simulink model "EMC_gaze"  (R2015a)
settings: Solver=ode4  SolverMode=MultiTasking  StartTime=0.0  StopTime=inf  FixedStep=BKIN_STEP_TIME  RelTol=1e-3
StartFcn:
  |  warndlg('Dexterit-E models cannot run under simulation. Please compile your model and run it from within Dexterit-E.');set_param(bdroot,'SimulationCommand','stop')
model workspace (MAT data in the model file):
  BKIN_KINEMATIC_FRAME_SIZE = 400
  BKIN_STEP_TIME = 0.00025
  COLOR = 4
  COL_X = 1
  COL_Y = 2
  E_NO_EVENT = 0
  LOAD_X = 1
  LOAD_Y = 2
  MOVEMENT_DELAY = 3
  PATH_LENGTH = 1
  PATH_PERIOD = 2
  POST_TRIAL_DELAY = 4
  RADIUS = 3
  TRAJECTORY = 1
  TRAJECTORY_TYPE = 2
  TRIAL_END = 3
  TRIAL_MOVEMENT = 2
  TRIAL_RESET = 4
  TRIAL_START = 1
  X_POSITION = 1
  Y_POSITION = 2
  col_x = 1
  col_y = 2
  ANGULAR_THRESHOLD = 5
  GAZE_EXIT = 6
  START_REACHED = 7
  FIXATION_DURATION = 6
  TRACKING_TARGET_ROW = 7
  FEEDBACK_COLOR = 5
  CROSS_LOGICAL_RADIUS = 8
  DETECT_FIXATION = 8
  GAZE_IN_TARGET = 5
  START_STABILIZATION = 9
  HAND_IN_TARGET = 9
  BACKGROUND_LOAD = 10
  DIST_BETWEEN_TRAJ = 11
  STRAIGHT_PAUSE_TIME = 12
libraries: simulink x14, xpcrtudplib x12, xpcutilitieslib x10, xpcobsoletelib x8, slrtlib x2, ethercat x2, General x2, Video x2, KINARM_EP_loads x1, KINARM_general x1
(part 5 of 7)

== matlab function EMC_gaze/DataLogging/Receive_Gaze/Embedded MATLAB Function1 ==
  data: input input; pupil_area_PIXELS input; tracking_status input; tracking_available input; camtheta input; camera_GLOBAL input; focal_length input; gazeXYCalculated output; head_data input; pupil_area_GLOBAL output; gaze_unit_vector_GLOBAL output; pupil_GLOBAL output; target_GLOBAL output
function [gazeXYCalculated, pupil_area_GLOBAL, gaze_unit_vector_GLOBAL, pupil_GLOBAL, target_GLOBAL] = fcn(input, pupil_area_PIXELS, tracking_status, tracking_available, camtheta,camera_GLOBAL, focal_length, head_data)

% The following are some details on the Eyelink camera
EL_target_distance_scaling_factor = 10000;					%target distance is reported by Eyelink in 1/10 of mm units
EL_pix_per_mm = 200;										%there are 200 pixels/mm on the Eyelink 1000 camera sensor

raw_pupil = [input(1) input(2)];
href = [input(3); input(4); 0];
target_distance_in = head_data(3);
%%%%%%%%%%%%%%%%%%%%%%%%%%%%%%%%%%
%% Tarkesh
target_position_in = head_data(1:2);
%%%%%%%%%%%%%%%%%%%%%%%%%%%%%%%%%%%%%%
target_distance = target_distance_in / EL_target_distance_scaling_factor;		% distance of the target from the camera (m)

%if there is a blink or other problem then send out errors. C3D file does not like NaN, so we output -100.
if tracking_status == 4 || tracking_available == 0 || (href(1) == 0 && href(2) == 0) || (raw_pupil(1) == -32768 && raw_pupil(2) == -32768)
    gazeXYCalculated = [-100; -100];
	pupil_area_GLOBAL = -100;
    gaze_unit_vector_GLOBAL = [-100; -100; -100];
    pupil_GLOBAL = [-100; -100; -100];
    target_GLOBAL = [-100; -100; -100];
    return
end

[Rx Ry Rz] = calc_R_from_angles(camtheta(1), camtheta(2), 0);
R_CMRA2GLBL = Rx * Ry;
%R_GLBL2CMRA = R_CMRA2GLBL';

%camera_GLOBAL_Trans = camera_GLOBAL';
pupil_XY_Sensor = convertPupilToSensor(raw_pupil(1), raw_pupil(2), EL_pix_per_mm);
[gaze_GLOBAL, pupil_GLOBAL] = calc_GAZE(pupil_XY_Sensor, target_distance, href, focal_length, camera_GLOBAL, R_CMRA2GLBL);
gazeXYCalculated = gaze_GLOBAL(1:2);

%%%%%%%%%%%%%%%%%%%%%%%%%%5
%% Tarkesh
target_XY_Sesor = convertPupilToSensor(target_position_in(1), target_position_in(2), EL_pix_per_mm);
[~, target_GLOBAL] = calc_GAZE(target_XY_Sesor, target_distance, href, focal_length, camera_GLOBAL, R_CMRA2GLBL);
%%%%%%%%%%%%%%%%%%%%%%%%%%

%%convert the pupil area from pixels on the sensor, to m^2, correcting for camera and gaze angle
% pupil area on the camera sensor, in m^2
pupil_area_SENSOR = pupil_area_PIXELS / ( (EL_pix_per_mm * 1000 ) ^ 2);		

% pupil area in the global workspace, projected onto a plane parallel to the camera sensor in m^2
pupil_area_GLOBAL_projection = pupil_area_SENSOR * (target_distance / focal_length) ^ 2; 

% create a unit vector that is normal to the camera sensor, in GLOBAL coordinates
sensor_unit_vector_GLOBAL = R_CMRA2GLBL * [0; 0; 1];

% create a unit vector for the subject's gaze
gaze_vector_GLOBAL = pupil_GLOBAL - gaze_GLOBAL;
gaze_unit_vector_GLOBAL = gaze_vector_GLOBAL / norm(gaze_vector_GLOBAL);

% calculate the cosine of the angle between the unit vectors for gaze and the camera sensor
cos_gaze_camera_angle = dot(sensor_unit_vector_GLOBAL, gaze_unit_vector_GLOBAL); 

% correct the pupil area to account for the angle of the eye relative to the camera sensor plane
% We assume that the pupil is circular. In the plane formed by the two vectors, the distance needs 
% to be scaled by cos(theta). In the perpendicular plane, there is no scaling. Hence we do NOT 
% square the cos(theta) and the area is only corrected for by 1 / cos(theta). 
pupil_area_GLOBAL = pupil_area_GLOBAL_projection / cos_gaze_camera_angle;

% % % % For testing
% % % gaze_camera_angle  = acos(cos_gaze_camera_angle) * 180/pi();
% % % HREF_angle = atan2( norm(href), 15000) * 180 / pi();
% % % testing = [pupil_area_SENSOR*1e6, pupil_area_GLOBAL_projection*1e6, pupil_area_GLOBAL*1e6, gaze_camera_angle, HREF_angle, cos_gaze_camera_angle];
% % % testing2 = [sensor_unit_vector_GLOBAL; gaze_unit_vector_GLOBAL];



%% Functions
function [gaze_est_GLOBAL, pupil_GLOBAL] = calc_GAZE(pupil_SENSOR, target_distance, HREF_HREF, focal_length, camera_GLOBAL, R_CMRA2GLBL)
    % This function estimates GAZE based on data from the Eyelink.  To be used
    % during 'running' of a task. 

    % Convert pupil location from Eyelink sensor frame to camera reference
    % frame with camera at origin and rotated to camera's angle (W-axis along
    % camera's point of view)  
    pupil_CAMERA = [pupil_SENSOR * target_distance / focal_length; target_distance];
    pupil_distance = norm(pupil_CAMERA);

    % Rotation matrix to convert from HREF coordinates to camera coordinates.
    % HREF z-axis is defined as ray from camera to pupil.
    R_HREF2CMRA = calc_R_from_vectors(pupil_CAMERA, [0; 0; 1]);

    % Convert the HREF from HREF coordinates to canera coordinates.  Scale,
    % then rotate. 
    HREF_CAMERA = R_HREF2CMRA * (HREF_HREF * pupil_distance / 15000);

    % Then convert pupil and HREF locations from camera frame to global frame
    % by rotating and then shifting origins. 
    pupil_GLOBAL = R_CMRA2GLBL * pupil_CAMERA + camera_GLOBAL';
    HREF_GLOBAL = R_CMRA2GLBL * HREF_CAMERA + camera_GLOBAL';

    % Find intersection of gaze_ray (from pupil to HREF) with the subject_display plane
    norm_vector = [0; 0; 1];		% In the KINARM VR setup, the Z-axis is defined as normal to the subject display
    point_on_plane = [0; 0; 0];		% In the KINARM VR setup, the origin is defined as on the subject display plane

    % display([pupil_GLOBAL HREF_GLOBAL])
    gaze_est_GLOBAL = plane_line_intersect(norm_vector, point_on_plane, pupil_GLOBAL, HREF_GLOBAL);

function pupil_XY_Sensor = convertPupilToSensor(pupilX, pupilY, pix_per_mm)
%         Returns the projection of the pupil on the camera sensor in meters, based on inputs in some raw unit (not pixels)

    % the following constants are from Jiye, email Nov 7, 2011
    LEFTDROP = 32;				%pixels dropped at left of sensor
    TOPDROP = 48;				%lines dropped at top of sensor
    const_x = 7*176;			%no idea what this is.  Maybe number of pixels???
    const_y = 4*184 + 188;		%no idea what this is.  Maybe number of pixels???

    % from Jiye. Not sure excatly what they are (probably camera center in pixels)
    cam_rot_cx = const_x / 2 + LEFTDROP;			
    cam_rot_cy = const_y / 2 +TOPDROP;

    hor = 30000;
    lor = -30000;
    hr = 0.9;
    lr = 0.1;
    ld = 50;
    hdx = 1200;		%hmmm almost same as const_x, which is 1232
    hdy = 920;		%hmmm almost same as const_y, which is 924

    scx = (hor-lor) / (hdx - ld) / (hr-lr);
    ofx = lor - (ld + (hdx - ld) * lr )* scx;

    scy = (hor-lor) / (hdy - ld) / (hr-lr);
    ofy = lor - (ld + (hdy - ld) * lr )* scy;

    % calculate the pupil in camera sensor coordinates (pixels)
    px = (pupilX - ofx) / scx;
    py = (pupilY - ofy) / scy;

    ppl_mmX = - ( (cam_rot_cx - px) / pix_per_mm );
    ppl_mmY =   ( (cam_rot_cy - py) / pix_per_mm );

    pupil_XY_Sensor = [ppl_mmX / 1000; ppl_mmY / 1000];
    
function [Rx Ry Rz] = calc_R_from_angles(xrot, yrot, zrot)
    % This function creates the three rotation matrices for rotations about the
    % x, y and z axes.  Input rotations are in degrees.

    xrot = xrot/180*pi;		%convert to radians
    yrot = yrot/180*pi;		%convert to radians
    zrot = zrot/180*pi;		%convert to radians
    Rx = [1 0 0; 0 cos(xrot) -sin(xrot); 0 sin(xrot) cos(xrot)]; 
    Ry = [cos(yrot) 0 sin(yrot); 0 1 0; -sin(yrot) 0 cos(yrot)]; 
    Rz = [cos(zrot) -sin(zrot) 0; sin(zrot) cos(zrot) 0 ; 0 0 1]; 

    
function R = calc_R_from_vectors(v1, v2)
    % This function calculates a rotation matrix, given two vectors, such that
    % the rotation matrix will rotate from v1 to v2.

    rot_axis = cross(v2, v1);			%axis that is perpendicular to the two vectors

    % If either of the vectors v1 or v2 is = [0 0 0], or if they are parallel
    % (i.e. norm(rot_axis) == 0), then there is no rotation.  But math errors
    % will occur, so we need to check for these cases.   
    if (norm(v1) == 0) || (norm(v2) == 0)	|| (norm(rot_axis) == 0)
        R = eye(3);																%identity matrix results in no rotation
    else
        rot_angle = asin( norm(rot_axis) / norm(v1) / norm(v2) );				%angle of rotation about rot_axis
        n = rot_axis / norm(rot_axis);											%normalize to get a unit vector for the rotation
        n_cross_product_matrix = [ 0 -n(3) n(2); n(3) 0 -n(1); -n(2) n(1) 0];	%def'n of cross product matrix
        cosA = cos(rot_angle);
        sinA = sin(rot_angle);
        R = eye(3) * cosA + sinA * n_cross_product_matrix + (1 - cosA) * (n * n');
    % 	display(rot_angle);
    end


function I = plane_line_intersect(n,V0,P0,P1)
    %plane_line_intersect computes the intersection of a plane and a segment(or
    %a straight line)
    % Inputs: 
    %       n: normal vector of the Plane 
    %       V0: any point that belongs to the Plane 
    %       P0: end point 1 of the segment P0P1
    %       P1:  end point 2 of the segment P0P1
    %
    %Outputs:
    %      I    is the point of interection 
    %     Check is (DELETED AND NOT USED HERE) an indicator:
    %      0 => disjoint (no intersection)
    %      1 => the plane intersects P0P1 in the unique point I
    %      2 => the segment lies in the plane
    %      3=>the intersection lies outside the segment P0P1
    %
    % Example:
    % Determine the intersection of following the plane x+y+z+3=0 with the segment P0P1:
    % The plane is represented by the normal vector n=[1 1 1]
    % and an arbitrary point that lies on the plane, ex: V0=[1 1 -5]
    % The segment is represented by the following two points
    % P0=[-5 1 -1]
    %P1=[1 2 3]   
    % [I,check]=plane_line_intersect([1 1 1],[1 1 -5],[-5 1 -1],[1 2 3]);

    %This function is written by :
    %                             Nassim Khaled
    %                             Wayne State University
    %                             Research Assistant and Phd candidate
    %If you have any comments or face any problems, please feel free to leave
    %your comments and i will try to reply to you as fast as possible.

    I=[0; 0; 0];
    u = P1-P0;
    w = P0 - V0;
    D = dot(n,u);
    N = -dot(n,w);
    check=0;
    if abs(D) < 10^-7        % The segment is parallel to plane
            if N == 0           % The segment lies in plane
                check=2;
                return
            else
                check=0;       %no intersection
                return
            end
    end

    %compute the intersection parameter
    sI = N / D;
    I = P0+ sI.*u;

== matlab function EMC_gaze/DataLogging/Receive_Gaze/clean_packet ==
  data: pack_in input; pack_out output; len_out output; len_in input
function [pack_out, len_out] = clean_packet(pack_in, len_in)

%for some reason, during calibration we can get very large packets that 
%blow up the c code for parsing the packets. If we get a large packet
%we can ignore it.

if len_in < 512
    pack_out = pack_in;
    len_out = len_in;
else
    pack_out = zeros(512, 1, 'uint8');
    len_out = int32(0);
end

== matlab function EMC_gaze/DataLogging/Receive_Gaze/convert to seconds2 ==
  data: event_data input; event_data_out output; start_time input; eyelink_timestamp input
function event_data_out = fcn(event_data, start_time, eyelink_timestamp)

persistent last_timestamp

if isempty(last_timestamp)
	last_timestamp = uint32(0);
end

%DEX-3313 if eyelink has stopped sending us data then we should not flood
%Dex with events.
if last_timestamp == eyelink_timestamp
	event_data_out = [0; 0; 0];
	return
end

last_timestamp = eyelink_timestamp;
event_data_out = event_data;

if event_data(1) ~= 0
    event_data_out(2) = (event_data(2) - start_time) / 1000.0;
    event_data_out(3) = (event_data(3) - start_time) / 1000.0;
end

== matlab function EMC_gaze/KINARM_EP_Apply_Loads/Remove_NaNs_and_Inf ==
  settings: fimath=|
      | fimath(...
      | 'RoundMode', 'floor',...
      | 'OverflowMode', 'wrap',...
      | 'ProductMode', 'KeepLSB', 'ProductWordLength', 32,...
      | 'SumMode', 'KeepLSB', 'SumWordLength', 32,...
      | 'CastBeforeSum', false)
  data: in input; out output
function out= fcn(in)

% This function removes all infinite and NaN values from the input.

out = zeros(size(in));		%default value of output

for ii = 1:length(in)
	if isfinite( in(ii) )	%only pass the input to the output if it is finite
		out(ii) = in(ii); 
	end
end

== matlab function EMC_gaze/KINARM_EP_Apply_Loads/Remove_NaNs_and_Inf1 ==
  settings: fimath=|
      | fimath(...
      | 'RoundMode', 'floor',...
      | 'OverflowMode', 'wrap',...
      | 'ProductMode', 'KeepLSB', 'ProductWordLength', 32,...
      | 'SumMode', 'KeepLSB', 'SumWordLength', 32,...
      | 'CastBeforeSum', false)
  data: in1 input; out output; in2 input; in3 input; in4 input
function out= fcn( in1,in2,in3,in4)

% This function removes all infinite and NaN values from the input.

out = [in1 in2 in3 in4];
if ~isfinite(in1)
    out(1) = 0;
end
if ~isfinite(in2)
    out(2) = 0;
end
if ~isfinite(in3)
    out(3) = 0;
end
if ~isfinite(in4)
    out(4) = 0;
end

== matlab function EMC_gaze/KINARM_EP_Apply_Loads/detect motor state/MATLAB Function ==
  data: motor_status input; motors_enabled output; grip_sensor input; is_ecat input
function motors_enabled = fcn(motor_status, grip_sensor, is_ecat)
%#codegen

motors_enabled = motor_status == 0 && (~is_ecat || grip_sensor == 1);

== matlab function EMC_gaze/KINARM_EP_Apply_Loads/detect motor state1/MATLAB Function ==
  data: motor_status input; motors_enabled output; grip_sensor input; is_ecat input
function motors_enabled = fcn(motor_status, grip_sensor, is_ecat)
%#codegen

motors_enabled = motor_status == 0 && (~is_ecat || grip_sensor == 1);

== matlab function EMC_gaze/DataLogging/Poll Force Plates/plate1/parse packet 1 ==
  data: packet input; forces output; moments output; timer output; calibration input; gain input; ain_slope input; ain_offset input; orientation input; zero_voltage input
function [forces, moments, timer] = fcn(packet, calibration, gain, ain_slope, ain_offset, orientation, zero_voltage)
    %This pulls voltages and timer infomation from the packet we got back from
    %the lab jack.
    
    voltages = zeros(1, 8);
    timers = zeros(1, 3);
    
    for n = 1:8
        bits = readUShort(packet, 13 + ((n - 1)*2));
        voltages(n) = binaryToCalibratedAnalogVoltage(bits, ain_slope, ain_offset);
    end
    
    for n = 1:3
        timers(n) = readUInt(packet, 53 + ((n - 1)*4));
    end
    
    %convert the time stamp to a time in seconds.
    timer = timers(1) / 750000.0; 
    
    %all voltages are between -2.5 to 2.5, here we are normalizeing what we read to zero.
    voltages = voltages - zero_voltage;
    voltages = voltages(1:8); % only the first 8 channels matter.
    
    %using the calibration matrix we convert the to the forces and moments
    values = calibration * (voltages / gain)';
    forces = values(1:3);
    moments = values(4:6);
    
	%reverse the Z force to get it into global coordinates.
	forces(3) = -forces(3);
	
	%considering the positions of the cables push all measures into global coordinates
    if orientation == 0
        forces(2) = -forces(2);
        moments(2) = -moments(2);
    elseif orientation == 90
        y = forces(2);
        forces(2) = -forces(1);
        forces(1) = -y;

        y = moments(2);
        moments(2) = -moments(1);
        moments(1) = -y;
	elseif orientation == 180
        forces(1) = -forces(1);        
        moments(1) = -moments(1);        
    elseif orientation == 270
        y = forces(2);
        forces(2) = forces(1);
        forces(1) = y;

		y = moments(2);
        moments(2) = moments(1);
        moments(1) = y;
    end
end

function val = readUShort(data, offset)
    p1 = uint32(data(offset));
    p2 = uint32(data(offset + 1));
    val = double(p1 + (p2 * 256));
end

function val = readUInt(data, offset)
    p1 = uint32(data(offset));
    p2 = uint32(data(offset + 1));
    p3 = uint32(data(offset + 2));
    p4 = uint32(data(offset + 3));
    val = double(p1 + (p2 * 256) + (p3 * 2^16) + (p4 * 2^24));
end

function voltage = binaryToCalibratedAnalogVoltage(bits, ain_slope, ain_offset)
    voltage = (bits * ain_slope) + ain_offset;
end

== matlab function EMC_gaze/DataLogging/Poll Force Plates/plate2/parse packet 1 ==
  data: packet input; forces output; moments output; timer output; calibration input; gain input; ain_slope input; ain_offset input; orientation input; zero_voltage input
function [forces, moments, timer] = fcn(packet, calibration, gain, ain_slope, ain_offset, orientation, zero_voltage)
    %This pulls voltages and timer infomation from the packet we got back from
    %the lab jack.
    
    voltages = zeros(1, 8);
    timers = zeros(1, 3);

    for n = 1:8
        bits = readUShort(packet, 13 + ((n - 1)*2));
        voltages(n) = binaryToCalibratedAnalogVoltage(bits, ain_slope, ain_offset);
    end
    
    for n = 1:3
        timers(n) = readUInt(packet, 53 + ((n - 1)*4));
    end
    
    %convert the time stamp to a time in seconds.
    timer = timers(1) / 750000.0; 
    
    %all voltages are between -2.5 to 2.5, here we are normalizeing what we read to zero.
    voltages = voltages - zero_voltage;
    voltages = voltages(1:8); % only the first 8 channels matter.
    
    %using the calibration matrix we convert the to the forces and moments
    values = calibration * (voltages / gain)';
    forces = values(1:3);
    moments = values(4:6);
    
	%reverse the Z force to get it into global coordinates.
	forces(3) = -forces(3);

	%considering the positions of the cables push all measures into global coordinates
    if orientation == 0
        forces(2) = -forces(2);
        moments(2) = -moments(2);
    elseif orientation == 90
        y = forces(2);
        forces(2) = -forces(1);
        forces(1) = -y;

        y = moments(2);
        moments(2) = -moments(1);
        moments(1) = -y;
	elseif orientation == 180
        forces(1) = -forces(1);        
        moments(1) = -moments(1);        
    elseif orientation == 270
        y = forces(2);
        forces(2) = forces(1);
        forces(1) = y;

		y = moments(2);
        moments(2) = moments(1);
        moments(1) = y;
    end
end

function val = readUShort(data, offset)
    p1 = uint32(data(offset));
    p2 = uint32(data(offset + 1));
    val = double(p1 + (p2 * 256));
end

function val = readUInt(data, offset)
    p1 = uint32(data(offset));
    p2 = uint32(data(offset + 1));
    p3 = uint32(data(offset + 2));
    p4 = uint32(data(offset + 3));
    val = double(p1 + (p2 * 256) + (p3 * 2^16) + (p4 * 2^24));
end

function voltage = binaryToCalibratedAnalogVoltage(bits, ain_slope, ain_offset)
    voltage = (bits * ain_slope) + ain_offset;
end

== matlab function EMC_gaze/DataLogging/Poll KINARM/Force Sensor Control/Force Sensor 1 Subsystem/Create timestamp ==
  data: times_in input; timestamp_out output
function timestamp_out = fcn(times_in)

persistent start_time
persistent last_time

if isempty(start_time)
   start_time = uint32(0);
end

if isempty(last_time)
    last_time = uint32(0);
end

if start_time == 0 && times_in(2) > 0
    start_time = times_in(2);
end

if times_in(2) < start_time
    start_time = -(last_time - start_time);
end

%F/T sensor clock runs at 7Khz according to the manual,
%using a 32 bit integer for this gives about 7 days before it will roll
%over. This means we need to account for roll overs in order to make
%analysis sane.
timestamp_out = double(times_in(2) - start_time) / 7000.0;
last_time = times_in(2);

== matlab function EMC_gaze/DataLogging/Poll KINARM/Force Sensor Control/Force Sensor 2 Subsystem/Create timestamp ==
  data: times_in input; timestamp_out output
function timestamp_out = fcn(times_in)

persistent start_time
persistent last_time

if isempty(start_time)
   start_time = uint32(0);
end

if isempty(last_time)
    last_time = uint32(0);
end

if start_time == 0 && times_in(2) > 0
    start_time = times_in(2);
end

if times_in(2) < start_time
    start_time = -(last_time - start_time);
end

%F/T sensor clock runs at 7Khz according to the manual,
%using a 32 bit integer for this gives about 7 days before it will roll
%over. This means we need to account for roll overs in order to make
%analysis sane.
timestamp_out = double(times_in(2) - start_time) / 7000.0;
last_time = times_in(2);

== matlab function EMC_gaze/DataLogging/Poll KINARM/PMAC Subsystem/read_pmac/DPRAM Access Subsystem/TypeCast ==
  data: u input; y output
function y = fcn(u)

% EML determines output class and size based on first usage
% for some reason the typecast is not setting it correctly, so we 
% explicitly define it first.
y = single(0);

% in order for the typecast to work, both temp and y must be 32 bit
temp = cast(u, 'uint32');
y = typecast(temp, 'single');

== matlab function EMC_gaze/DataLogging/Poll KINARM/PMAC Subsystem/read_pmac/Monitor_status ==
  data: status_data input; servo_counter input; robotCount input; force_scale output; plcc_version input
function force_scale = monitor_system_status(status_data, servo_counter, robotCount, plcc_version)

persistent no_update_count;
persistent last_servo_counter;

if isempty(no_update_count)
   no_update_count = 0;
end

if isempty(last_servo_counter)
    last_servo_counter = uint32(0);
end

pmac_fault_state = uint32(status_data(2));
plcc_switch = status_data(3);
force_scale = 1;

%plcc versions >1000 are custom
if plcc_version >= 6.0 && plcc_version < 1000
    %if the task is running and the servo amp counter is not
    if plcc_switch == 4.0 && last_servo_counter == servo_counter
        no_update_count = no_update_count + 1;    
        %after 5 cycles with the counter not running we should kill forces.
        if no_update_count >= 5
            force_scale = 0;
        end
    else
        no_update_count = 0;
    end
    last_servo_counter = servo_counter; 
end

%plcc versions >1000 are custom
if plcc_version >= 7.0 && plcc_version < 1000
    %if it is unilateral and the robot state is faulted then kill the forces
    if robotCount == 1 && bitand(pmac_fault_state, 1) == 1
        force_scale = 0;
    %if the system is bilateral and either robot is faulted, kill forces.
    elseif robotCount == 2 && bitand(pmac_fault_state, 3) ~= 0
        force_scale = 0;
    end
end

if plcc_version == 0
    force_scale = 0;
end

== matlab function EMC_gaze/DataLogging/Poll KINARM/PMAC Subsystem/read_pmac/Robot_data_builder ==
  data: bR1HasSecondardy input; bR2HasSecondardy input; robot1Data input; robot2Data input; robot1PrimaryEncData input; robot2PrimaryEncData input; robot1DataOut output; robot2DataOut output; servoCounter input; plccVer input; robot1PrimaryEncDataOut output; robot2PrimaryEncDataOut output
function [robot1DataOut, robot2DataOut, robot1PrimaryEncDataOut, robot2PrimaryEncDataOut] = convertPMACValues(bR1HasSecondardy, bR2HasSecondardy, robot1Data, robot2Data, robot1PrimaryEncData, robot2PrimaryEncData, servoCounter, plccVer)

    persistent robot1Struct robot2Struct robot1StructPrimary robot2StructPrimary servoValuesR1 servoValuesR2
    
    if isempty(robot1Struct)
        robot1Struct = getStruct();
        robot2Struct = getStruct();
        robot1StructPrimary = getStruct();
        robot2StructPrimary = getStruct();
        servoValuesR1 = zeros(5, 1);
        servoValuesR2 = zeros(5, 1);
    end
    
    if plccVer < 7
        robot1DataOut = robot1Data;
        robot2DataOut = robot2Data;
        robot1PrimaryEncDataOut = robot1PrimaryEncData;
        robot2PrimaryEncDataOut = robot2PrimaryEncData;
        return
    end
    
    if servoCounter(1) ~= servoValuesR1(1)
        robot1Struct = updatePositions(robot1Struct, robot1Data, bR1HasSecondardy);
        robot1StructPrimary = updatePositions(robot1StructPrimary, robot1PrimaryEncData, 0);
        servoValuesR1 = insertVal(servoValuesR1, servoCounter(1));
        robot1Struct = calculateVelAcc(robot1Struct, servoValuesR1, robot1Data);
        robot1StructPrimary = calculateVelAcc(robot1StructPrimary, servoValuesR1, robot1PrimaryEncData);
    end
    
    if servoCounter(2) ~= servoValuesR2(1)
        robot2Struct = updatePositions(robot2Struct, robot2Data, bR2HasSecondardy);
        robot2StructPrimary = updatePositions(robot2StructPrimary, robot2PrimaryEncData, 0);
        servoValuesR2 = insertVal(servoValuesR2, servoCounter(2));
        robot2Struct = calculateVelAcc(robot2Struct, servoValuesR2, robot2Data);
        robot2StructPrimary = calculateVelAcc(robot2StructPrimary, servoValuesR2, robot2PrimaryEncData);
    end
    
    robot1DataOut = insertVelAcc(robot1Data, robot1Struct);
    robot2DataOut = insertVelAcc(robot2Data, robot2Struct);

    robot1PrimaryEncDataOut = insertVelAcc(robot1PrimaryEncData, robot1StructPrimary);
    robot2PrimaryEncDataOut = insertVelAcc(robot2PrimaryEncData, robot2StructPrimary);
    
    %We used to provide a filtered velocity, but we can't with EtherCAT and
    %it was not being used anywhere anyway. 
    robot1DataOut(7:8) = robot1DataOut(3:4);
    robot2DataOut(7:8) = robot2DataOut(3:4);
end


function robotDataOut = insertVelAcc(robotData, robotStruct)
    robotDataOut = robotData(:);
    robotDataOut(3) = robotStruct.shoVel(1);
    robotDataOut(4) = robotStruct.elbVel(1);
    robotDataOut(5) = robotStruct.shoAcc;
    robotDataOut(6) = robotStruct.elbAcc;
end

function st=getStruct()
    st = struct('shoPos', zeros(5, 1), 'elbPos', zeros(5, 1), ...
        'shoVel', zeros(5, 1), 'elbVel', zeros(5, 1), ...
        'shoAcc', 0, 'elbAcc', 0, 'bHasSecondary', 0);
end

function robotStruct = updatePositions(robotStruct, robotData, bHasSecondardy)
    robotStruct.shoPos = insertVal(robotStruct.shoPos, robotData(1));
    robotStruct.elbPos = insertVal(robotStruct.elbPos, robotData(2));
    robotStruct.bHasSecondary = bHasSecondardy;
end

function arr=insertVal(arr, v)
    arr = circshift(arr, 1);
    arr(1) = v;
end

function robotStructOut=calculateVelAcc(robotStruct, servoValues, robotData)
    %matches from PMAC code
    robotStructOut = robotStruct;
    servoTimeStep = (7427414.0/8388608.0) / 1000; 
    %do not name this anything that will make it the first variable name in
    %this method alphabetically. Seriously. With the name "duration" compiling
    %a model would work in 2010a, but nothing higher. Most models would compile,
    %but the verification task would not!
    stepDuration = 0;
    
    if robotStruct.bHasSecondary
        stepDuration = ((servoValues(1) - servoValues(2)) * servoTimeStep);
        if stepDuration == 0
            shoVel = robotStruct.shoVel(1);
            elbVel = robotStruct.elbVel(1);
        else
            shoVel = (robotStruct.shoPos(1) - robotStruct.shoPos(2)) / stepDuration;
            elbVel = (robotStruct.elbPos(1) - robotStruct.elbPos(2)) / stepDuration;        
        end
    else
        shoVel = robotData(3);
        elbVel = robotData(4);
    end
    
    robotStructOut.shoVel = insertVal(robotStruct.shoVel, shoVel);
    robotStructOut.elbVel = insertVal(robotStruct.elbVel, elbVel);

    if robotStruct.bHasSecondary        
        if stepDuration == 0
            shoAcc = robotStruct.shoAcc;
            elbAcc = robotStruct.elbAcc;
        else
            shoAcc = (robotStruct.shoVel(1) - robotStruct.shoVel(2)) / stepDuration;
            elbAcc = (robotStruct.elbVel(1) - robotStruct.elbVel(2)) / stepDuration;        
        end
    else
        stepDuration = ((servoValues(1) - servoValues(5)) * servoTimeStep);
        shoAcc = (robotStruct.shoVel(1) - robotStruct.shoVel(5)) / stepDuration;
        elbAcc = (robotStruct.elbVel(1) - robotStruct.elbVel(5)) / stepDuration;        
    end    
    
    robotStructOut.shoAcc = shoAcc;
    robotStructOut.elbAcc = elbAcc;
end

== matlab function EMC_gaze/DataLogging/Poll KINARM/PMAC Subsystem/read_pmac/filter_velocities ==
  data: robot1Data input; robot2Data input; robot1DataOut output; robot2DataOut output; servoCounters input; plccVer input
function [robot1DataOut, robot2DataOut] = filterVelocities(robot1Data, robot2Data, servoCounters, plccVer)

    persistent robot1Struct robot2Struct
    POLES = 2;
    
    if isempty(robot1Struct)
        robot1Struct = getStruct(POLES);
        robot2Struct = getStruct(POLES);
    end
    
    if plccVer < 7
        robot1DataOut = robot1Data;
        robot2DataOut = robot2Data;
        return
    end
    
    robot1DataOut = robot1Data(:);
    robot2DataOut = robot2Data(:);
    
    robot1Struct = updateValues(robot1Struct, robot1Data, servoCounters(1), POLES);
    robot2Struct = updateValues(robot2Struct, robot2Data, servoCounters(2), POLES);
        
    %We used to provide a filtered velocity, but we can't with EtherCAT and
    %it was not being used anywhere anyway. 
    robot1DataOut(7:8) = [robot1Struct.shoVelFilt(POLES + 1), robot1Struct.elbVelFilt(POLES + 1)];
    robot2DataOut(7:8) = [robot2Struct.shoVelFilt(POLES + 1), robot2Struct.elbVelFilt(POLES + 1)];
end


function st=getStruct(poles)
    valueCount = poles + 1;
    st = struct('shoVel', zeros(valueCount, 1), 'elbVel', zeros(valueCount, 1), ...
        'shoVelFilt', zeros(valueCount, 1), 'elbVelFilt', zeros(valueCount, 1), ...
        'servoCounter', zeros(valueCount, 1));
end

function arr=insertVal(arr, v)
    arr = circshift(arr, -1);
    arr(length(arr)) = v;
end

function robotStruct = updateValues(robotStruct, robotData, servoCounter, POLES)
    if servoCounter == robotStruct.servoCounter(POLES + 1)
        return
    end
    
    robotStruct.servoCounter = insertVal(robotStruct.servoCounter, servoCounter);
    
    [robotStruct.shoVel, robotStruct.shoVelFilt] = filterJoint(robotStruct.shoVel, robotStruct.shoVelFilt, robotData(3), POLES);
    [robotStruct.elbVel, robotStruct.elbVelFilt] = filterJoint(robotStruct.elbVel, robotStruct.elbVelFilt, robotData(4), POLES);
end

function [velocitiesOut, velFilt] = filterJoint(velocities, filtVelocities, newVelocity, POLES)

%all filter constants from http://www-users.cs.york.ac.uk/~fisher/cgi-bin/mkfscript

    %GAIN = 4.143204922e+03; % 1KHz gain
    GAIN = 1.342624471e+03; %1.129 KHz gain (PMAC speed)
    
    %FILTER_VALUES = [-0.9565436765, 1.9555782403]; % 1KHz
    FILTER_VALUES = [-0.9243128082, 1.9213335686]; % 1.129 KHz
    
    velocitiesOut = insertVal(velocities, newVelocity / GAIN);
    velFilt = insertVal(filtVelocities, 0);

    velFilt(POLES + 1) = velocitiesOut(1) + ...
         velocitiesOut(2) * 2.0 + ...
         velocitiesOut(3) + ...
         velFilt(1) * FILTER_VALUES(1) + ...
         velFilt(2) * FILTER_VALUES(2);
    
     if isnan(velFilt(POLES + 1)) || isinf(velFilt(POLES + 1))
         velFilt(POLES + 1) = 0;
    end
end

== matlab function EMC_gaze/DataLogging/Poll KINARM/PMAC Subsystem/update settings/update status format ==
  data: pmacStatus input; outStatus output
function outStatus = fcn(pmacStatus)
%#eml

outStatus = zeros(1, 7, 'uint32');
outStatus(5:6) = pmacStatus(2:3);

STATUS_FUNCTIONING = uint32(0);
STATUS_READY = uint32(1);
STATUS_FAULTED = uint32(2);

%Each motor has 2 possible states: 0 working, 1 faulted. The READY state is only used by EtherCAT
for n=0:3
    motor = bitand( bitshift(pmacStatus(1), -n), 1);
    if motor == 1
       outStatus(n + 1) =  STATUS_FAULTED;
    else
        outStatus(n + 1) = STATUS_FUNCTIONING;
    end
end

== matlab function EMC_gaze/DataLogging/Poll KINARM/bkin_internal_testing/Data receive/MATLAB Function ==
  data: r1ShoElb input; kinematics output; r2ShoElb input; primary output; is_new_data input; clock_tick input; BKIN_STEP_TIME parameter
function [kinematics, primary] = fcn(r1ShoElb, r2ShoElb, is_new_data, clock_tick, BKIN_STEP_TIME)
%#codegen

persistent r1Sho r1Elb r2Sho r2Elb last_tick

if isempty(r1Sho)
   r1Sho = zeros(4, 1); 
   r1Elb = zeros(4, 1); 
   r2Sho = zeros(4, 1); 
   r2Elb = zeros(4, 1); 
   last_tick = zeros(4, 1);
end

if is_new_data > 0
    r1Sho(2:4) = r1Sho(1:3);
    r1Elb(2:4) = r1Elb(1:3);
    r2Sho(2:4) = r2Sho(1:3);
    r2Elb(2:4) = r2Elb(1:3);

    r1Sho(1) = r1ShoElb(1);
    r1Elb(1) = r1ShoElb(2);
    r2Sho(1) = r2ShoElb(1);
    r2Elb(1) = r2ShoElb(2);
    
    last_tick(2:4) = last_tick(1:3);
    last_tick(1) = double(clock_tick) * BKIN_STEP_TIME;
end

kinematics = zeros(20, 1);
primary = zeros(12, 1);

kinematics(1:2) = [r1Sho(1) r1Elb(1)];
%[kinematics(3), kinematics(5)] = velAndAcc(r1Sho, last_tick);
%[kinematics(4), kinematics(6)] = velAndAcc(r1Elb, last_tick);
%kinematics(7:8) = kinematics(5:6);

kinematics(11:12) = [r2Sho(1) r2Elb(1)];
%[kinematics(13), kinematics(15)] = velAndAcc(r2Sho, last_tick);
%[kinematics(14), kinematics(16)] = velAndAcc(r2Elb, last_tick);
%kinematics(17:18) = kinematics(15:16);

primary(1:6) = kinematics(1:6);
primary(7:12) = kinematics(11:16);
end

function [vel, acc] = velAndAcc(values, times)
    vel_diff1 = diff(values);
    time_diff1 = diff(times);
    vel = mean(vel_diff1 ./ time_diff1);

    vel_diff2 = diff(vel_diff1);
    time_diff2 = diff(time_diff1);
    acc = mean (vel_diff2 ./ time_diff2);
end

== matlab function EMC_gaze/DataLogging/Poll KINARM/constants/arm1/decode robot ==
  data: system_type input; robot_type input; isEP output; robot_version input; isHumanEXO output; isNHPEXO output; isClassicExo output; isUTSEXO output; isPMAC output; isECAT output
function [isEP, isHumanEXO, isNHPEXO, isClassicExo, isUTSEXO, isPMAC, isECAT] = fcn(system_type, robot_type, robot_version)
%#eml
isEP = 0;
isHumanEXO = 0;
isNHPEXO = 0;
isClassicExo = 0;
isUTSEXO = 0;
isPMAC = 0;
isECAT = 0;

if robot_type == 0
    isHumanEXO = 1;    
    if robot_version == 1
        isClassicExo = 1;        
    elseif robot_version == 2
        isUTSEXO = 1;
    end    
elseif robot_type == 1
    isEP = 1;
elseif robot_type == 2
    isNHPEXO = 1;        
    if robot_version == 1
        isClassicExo = 1;        
    elseif robot_version == 2
        isUTSEXO = 1;
    end
end

if system_type == 1
   isPMAC = 1;
elseif system_type == 2
    isECAT = 1;
end

== matlab function EMC_gaze/DataLogging/Poll KINARM/constants/arm2/decode robot ==
  data: system_type input; robot_type input; isEP output; robot_version input; isHumanEXO output; isNHPEXO output; isClassicExo output; isUTSEXO output; isPMAC output; isECAT output
function [isEP, isHumanEXO, isNHPEXO, isClassicExo, isUTSEXO, isPMAC, isECAT] = fcn(system_type, robot_type, robot_version)
%#eml
isEP = 0;
isHumanEXO = 0;
isNHPEXO = 0;
isClassicExo = 0;
isUTSEXO = 0;
isPMAC = 0;
isECAT = 0;

if robot_type == 0
    isHumanEXO = 1;    
    if robot_version == 1
        isClassicExo = 1;        
    elseif robot_version == 2
        isUTSEXO = 1;
    end    
elseif robot_type == 1
    isEP = 1;
elseif robot_type == 2
    isNHPEXO = 1;        
    if robot_version == 1
        isClassicExo = 1;        
    elseif robot_version == 2
        isUTSEXO = 1;
    end
end

if system_type == 1
   isPMAC = 1;
elseif system_type == 2
    isECAT = 1;
end

== stateflow chart EMC_gaze/DataLogging/Poll KINARM/control read write ==
  settings: sampleTime=0.0005
  state RunSim/
    during:
    bkin_testing;
    buildKINData
  state RunECat/
    during:
    ecat;
    buildKINData;
  state RunPMAC/
    during:
    pmac;
    buildKINData;
  (default) -> (junction 216)
  (junction 216) -> RunSim [order 3]
  (junction 216) -> RunPMAC [order 2] : [system_type == 1]
  (junction 216) -> RunECat [order 1] : [system_type == 2]
  data: system_type input double
  events: bkin_testing output FUNCTION_CALL_EVENT; ecat output FUNCTION_CALL_EVENT; pmac output FUNCTION_CALL_EVENT; buildKINData output FUNCTION_CALL_EVENT
